simulink model "wec_reinforcementlearningcopy"  (R2017b)
settings: Solver=VariableStepAuto  StartTime=0.0  StopTime=900  RelTol=1e-3
values from neighbouring files (symbols this model uses):
  A1 = 3.3e5    (= 330000)    [CS533DQN_FunctionApproximation.m]
  B1 = 9.7e4    (= 97000)    [CS533DQN_FunctionApproximation.m]
  B2 = action(action_idx,1)    [CS533DQN_FunctionApproximation.m]    (also in SIMULATOR.m = B2*9.7e4)
  K1 = 8.8e5    (= 880000)    [CS533DQN_FunctionApproximation.m]
  K2 = action(action_idx,2)    [CS533DQN_FunctionApproximation.m]    (also in SIMULATOR.m = K2*8.8e5)
undefined symbols (not defined in the file or in its folder): A2, dzb_0, wecControlLaw, wecRealPlant, wp, zb_0
settings Model: Creator=brekken  LastModifiedBy=ghleila
settings CodeAppCC: StateflowObjectComments=on

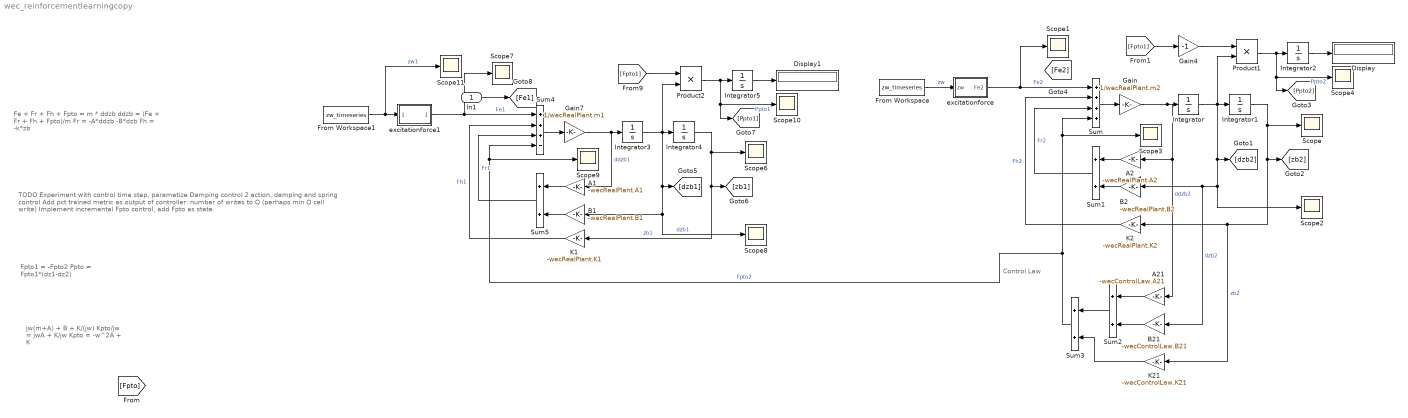
== system wec_reinforcementlearningcopy ==
  note: Fpto1 = -Fpto2
      | Ppto = Fpto1*(dz1-dz2)
  note: TODO
      |
      | Experiment with control time step, parametize
      | Damping control
      | 2 action, damping and spring control
      | Add pct trained metric as output of controller: number of writes to Q (perhaps min Q cell write)
      | Implement incremental Fpto control, add Fpto as state
  note: jw(m+A) + B + K/(jw)
      |
      | Kpto/jw = jwA + K/jw
      | Kpto = -w^2A + K
  note: Fe + Fr + Fh + Fpto = m * ddzb
      | ddzb = (Fe + Fr + Fh + Fpto)/m
      |
      | Fr = -A*ddzb -B*dzb
      |
      | Fh = -k*zb
  note: Control Law
  In1 : Inport
  A1 : Gain  Gain=-wecRealPlant.A1
  A2 : Gain  Gain=-wecRealPlant.A2
  A21 : Gain  Gain=-wecControlLaw.A21
  B1 : Gain  Gain=-wecRealPlant.B1
  B2 : Gain  Gain=-wecRealPlant.B2
  B21 : Gain  Gain=-wecControlLaw.B21
  Display : Display
  Display1 : Display
  From Workspace : FromWorkspace  VariableName=zw_timeseries  SampleTime=0  OutputAfterFinalValue=Setting to zero
  From Workspace1 : FromWorkspace  VariableName=zw_timeseries  SampleTime=0  OutputAfterFinalValue=Setting to zero
  Gain : Gain  Gain=1/wecRealPlant.m2
  Gain4 : Gain  Gain=-1
  Gain7 : Gain  Gain=1/wecRealPlant.m1
  Integrator : Integrator  InitialCondition=dzb_0
  Integrator1 : Integrator  InitialCondition=zb_0
  Integrator2 : Integrator
  Integrator3 : Integrator  InitialCondition=dzb_0
  Integrator4 : Integrator  InitialCondition=zb_0
  Integrator5 : Integrator
  K1 : Gain  Gain=-wecRealPlant.K1
  K2 : Gain  Gain=-wecRealPlant.K2
  K21 : Gain  Gain=-wecControlLaw.K21
  Product1 : Product
  Product2 : Product
  Scope{,1..4,6..11} (11 alike) : Scope
  Sum : Sum  Inputs=++++
  Sum{1..3,5} (4 alike) : Sum
  Sum4 : Sum  Inputs=+++-
  excitationforce : Subsystem
  excitationforce1 : Subsystem
  wires:
  B1/1 -> Sum5/2
  Product1/1 -> Scope4/1, [Ppto2], Integrator2/1  "Ppto2"
  Sum2/1 -> Sum3/1
  Gain/1 -> A2/1, A21/1, Integrator/1  "ddzb2"
  K1/1 -> Sum4/2  "Fh1"
  Integrator4/1 -> Scope6/1, [zb1], K1/1  "zb1"
  B21/1 -> Sum2/2
  Sum3/1 -> Scope9/1, Sum4/4, Scope3/1, Sum/4  "Fpto2"
  Product2/1 -> Scope10/1, [Ppto1], Integrator5/1  "Ppto1"
  Gain7/1 -> A1/1, Integrator3/1  "ddzb1"
  A1/1 -> Sum5/1
  Sum1/1 -> Sum/3  "Fr2"
  Sum/1 -> Gain/1
  A21/1 -> Sum2/1
  A2/1 -> Sum1/1
  B2/1 -> Sum1/2
  Integrator2/1 -> Display/1
  [Fpto1] -> Gain4/1
  Integrator1/1 -> Scope/1, [zb2], K21/1, K2/1  "zb2"
  Sum4/1 -> Gain7/1
  Integrator3/1 -> Product2/2, [dzb1], Scope8/1, B1/1, Integrator4/1  "dzb1"
  K21/1 -> Sum3/2
  K2/1 -> Sum/2  "Fh2"
  excitationforce/1(Fe2) -> Scope1/1, Sum/1  "Fe2"
  From Workspace1/1 -> Scope11/1, excitationforce1/1(zw1)  "zw1"
  Integrator/1 -> Product1/2, [dzb2], Scope2/1, B21/1, B2/1, Integrator1/1  "dzb2"
  From Workspace/1 -> excitationforce/1(zw)  "zw"
  In1/1 -> [Fe1]
  Gain4/1 -> Product1/1
  excitationforce1/1(Fe1) -> Scope7/1, Sum4/1  "Fe1"
  [Fpto1] -> Product2/1
  Integrator5/1 -> Display1/1
  Sum5/1 -> Sum4/3  "Fr1"

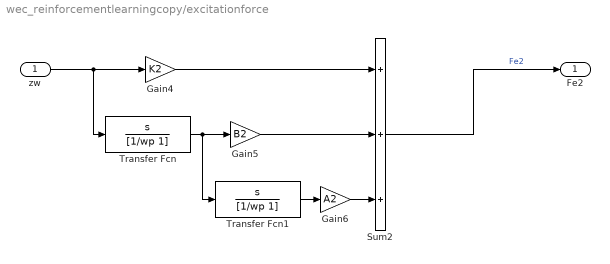
== system wec_reinforcementlearningcopy/excitationforce ==
  zw : Inport
  Gain4 : Gain  Gain=K2
  Gain5 : Gain  Gain=B2
  Gain6 : Gain  Gain=A2
  Sum2 : Sum  Inputs=+++
  Transfer Fcn : TransferFcn  Numerator=[1 0]  Denominator=[1/wp 1]
  Transfer Fcn1 : TransferFcn  Numerator=[1 0]  Denominator=[1/wp 1]
  Fe2 : Outport
  wires:
  Transfer Fcn/1 -> Transfer Fcn1/1, Gain5/1
  Gain5/1 -> Sum2/2
  Gain6/1 -> Sum2/3
  Sum2/1 -> Fe2/1  "Fe2"
  zw/1 -> Transfer Fcn/1, Gain4/1
  Transfer Fcn1/1 -> Gain6/1
  Gain4/1 -> Sum2/1

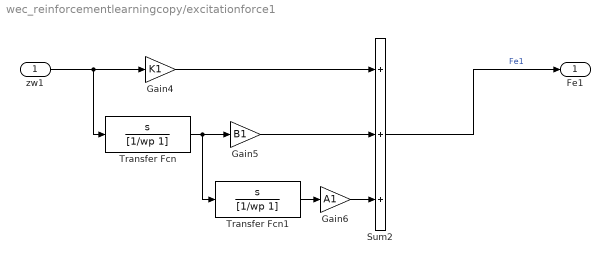
== system wec_reinforcementlearningcopy/excitationforce1 ==
  zw1 : Inport
  Gain4 : Gain  Gain=K1
  Gain5 : Gain  Gain=B1
  Gain6 : Gain  Gain=A1
  Sum2 : Sum  Inputs=+++
  Transfer Fcn : TransferFcn  Numerator=[1 0]  Denominator=[1/wp 1]
  Transfer Fcn1 : TransferFcn  Numerator=[1 0]  Denominator=[1/wp 1]
  Fe1 : Outport
  wires:
  Transfer Fcn/1 -> Transfer Fcn1/1, Gain5/1
  Gain5/1 -> Sum2/2
  Gain6/1 -> Sum2/3
  Sum2/1 -> Fe1/1  "Fe1"
  zw1/1 -> Transfer Fcn/1, Gain4/1
  Transfer Fcn1/1 -> Gain6/1
  Gain4/1 -> Sum2/1
